simulink model "testHarness"  (R2014b)
settings: Solver=ode15s  StartTime=0.0  StopTime=simTime  RelTol=1e-3
undefined symbols (not defined in the file): amplitude, c1, c11, c12, c13, c14, c15, c16, c17, c18, c19, c2, c20, c21, c22, c23, c24, c25, c3, c4, c5, c6, c7, c8, c9, en_speed
settings Model: Creator=xjin  LastModifiedBy=xjin
settings DataIOCC: LimitDataPoints=off
settings DebuggingCC: UnderspecifiedInitializationDetection=Classic  MergeDetectMultiDrivingBlocksExec=none

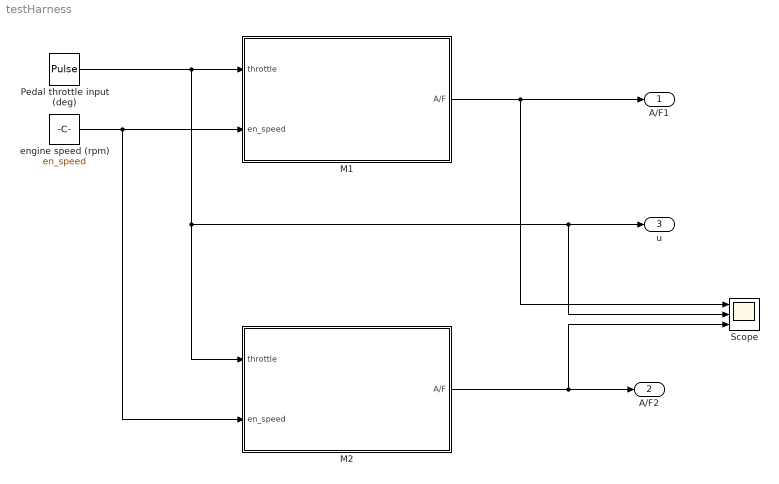
== system testHarness ==
  "M1 " : Subsystem
  M2 : Subsystem
  Pedal throttle input (deg) : DiscretePulseGenerator  PulseType=Time based  Amplitude=amplitude  Period=10  PulseWidth=50  PhaseDelay=3
  Scope : Scope  NumInputPorts=3
      settings: YMin=-5~-5~-5  YMax=5~5~5
  engine speed (rpm) : Constant  Value=en_speed
  A/F1 : Outport
  A/F2 : Outport  Port=2
  u : Outport  Port=3
  wires:
  "M1 "/1(A/F) -> Scope/1, A/F1/1
  engine speed (rpm)/1 -> M2/2(en_speed), "M1 "/2(en_speed)
  Pedal throttle input (deg)/1 -> "M1 "/1(throttle), M2/1(throttle), Scope/2, u/1
  M2/1(A/F) -> Scope/3, A/F2/1

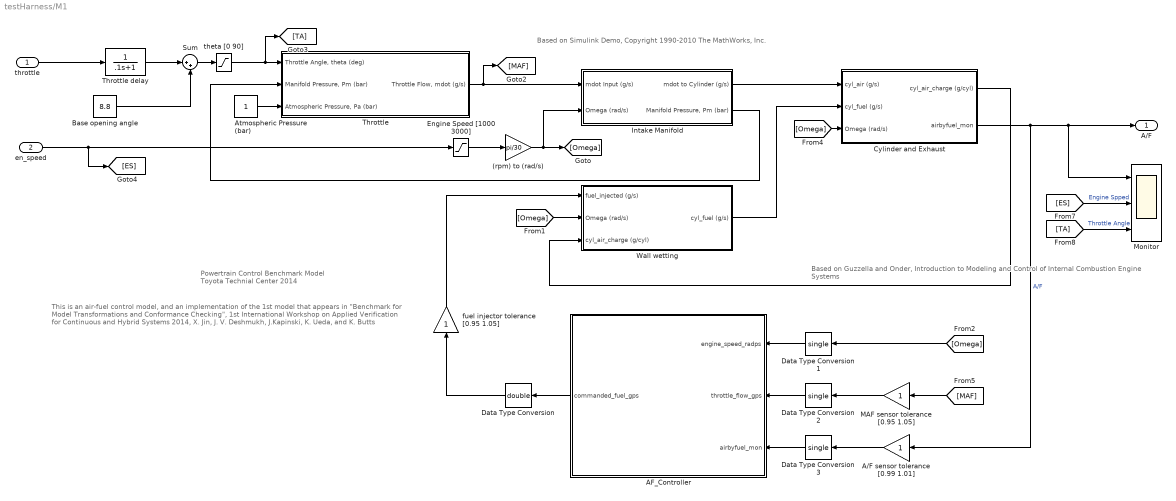
== system testHarness/M1  ==
  note: This is an air-fuel control model, and an implementation of the 1st model that appears in
      | "Benchmark for Model Transformations and Conformance Checking",
      | 1st International Workshop on Applied Verification for Continuous and Hybrid Systems 2014,
      | X. Jin, J. V. Deshmukh, J.Kapinski, K. Ueda, and K. Butts
  note: Powertrain Control Benchmark Model
      | Toyota Technial Center
      | 2014
  note: Based on Simulink Demo, Copyright 1990-2010 The MathWorks, Inc.
  note: Based on Guzzella and Onder, Introduction to Modeling and Control of Internal Combustion Engine Systems
  throttle : Inport
  en_speed : Inport  Port=2
  (rpm) to (rad/s) : Gain  Gain=pi/30
  A/F sensor tolerance [0.99 1.01] : Gain
  AF_Controller : Subsystem  TreatAsAtomicUnit=on
  Atmospheric Pressure (bar) : Constant
  Base opening angle : Constant  Value=8.8
  Cylinder and Exhaust : Subsystem
  Data Type Conversion : DataTypeConversion  OutDataTypeStr=double
  Data Type Conversion1 : DataTypeConversion  OutDataTypeStr=single
  Data Type Conversion2 : DataTypeConversion  OutDataTypeStr=single
  Data Type Conversion3 : DataTypeConversion  OutDataTypeStr=single
  Engine Speed [1000 3000] : Saturate  UpperLimit=3000  LowerLimit=1000
  Intake Manifold : Subsystem
  MAF sensor tolerance [0.95 1.05] : Gain
  Monitor : Scope  NumInputPorts=3
      settings: TimeRange=50  YMin=12.5~2850~5  YMax=20.5~3150~90
  Sum : Sum  Inputs=|++
  Throttle : Subsystem
  Throttle delay : TransferFcn  Denominator=[.1 1]
  Wall wetting : Subsystem
  fuel injector tolerance [0.95 1.05] : Gain
  theta [0 90] : Saturate  UpperLimit=90  LowerLimit=0
  A/F : Outport
  wires:
  (rpm) to (rad/s)/1 -> Intake Manifold/2(Omega (rad/s)), [Omega]
  Data Type Conversion/1 -> fuel injector tolerance [0.95 1.05]/1
  theta [0 90]/1 -> Throttle/1("Throttle Angle, theta (deg)"), [TA]
  Engine Speed [1000 3000]/1 -> (rpm) to (rad/s)/1
  Cylinder and Exhaust/2("airbyfuel_mon ") -> A/F sensor tolerance [0.99 1.01]/1, A/F/1, Monitor/1  "A/F"
  Data Type Conversion2/1 -> AF_Controller/2(throttle_flow_gps)
  Data Type Conversion3/1 -> AF_Controller/3(airbyfuel_mon)
  A/F sensor tolerance [0.99 1.01]/1 -> Data Type Conversion3/1
  [MAF] -> MAF sensor tolerance [0.95 1.05]/1
  Throttle/1("Throttle Flow, mdot (g/s)") -> [MAF], Intake Manifold/1(mdot Input (g/s))
  Intake Manifold/2("Manifold Pressure, Pm (bar)") -> Throttle/2("Manifold Pressure, Pm (bar)")
  Atmospheric Pressure (bar)/1 -> Throttle/3("Atmospheric Pressure, Pa (bar) ")
  Intake Manifold/1(mdot to Cylinder (g/s)) -> Cylinder and Exhaust/1(cyl_air (g/s))
  [Omega] -> Cylinder and Exhaust/3(Omega (rad/s))
  [Omega] -> Wall wetting/2(Omega (rad/s))
  Cylinder and Exhaust/1(cyl_air_charge (g/cyl)) -> Wall wetting/3(cyl_air_charge (g/cyl))
  [Omega] -> Data Type Conversion1/1
  fuel injector tolerance [0.95 1.05]/1 -> Wall wetting/1(fuel_injected (g/s))
  MAF sensor tolerance [0.95 1.05]/1 -> Data Type Conversion2/1
  AF_Controller/1(commanded_fuel_gps) -> Data Type Conversion/1
  Data Type Conversion1/1 -> AF_Controller/1(engine_speed_radps)
  Throttle delay/1 -> Sum/1
  Base opening angle/1 -> Sum/2
  Sum/1 -> theta [0 90]/1
  throttle/1 -> Throttle delay/1
  en_speed/1 -> [ES], Engine Speed [1000 3000]/1
  Wall wetting/1(cyl_fuel (g/s)) -> Cylinder and Exhaust/2(cyl_fuel (g/s))
  [TA] -> Monitor/3  "Throttle Angle"
  [ES] -> Monitor/2  "Engine Spped"

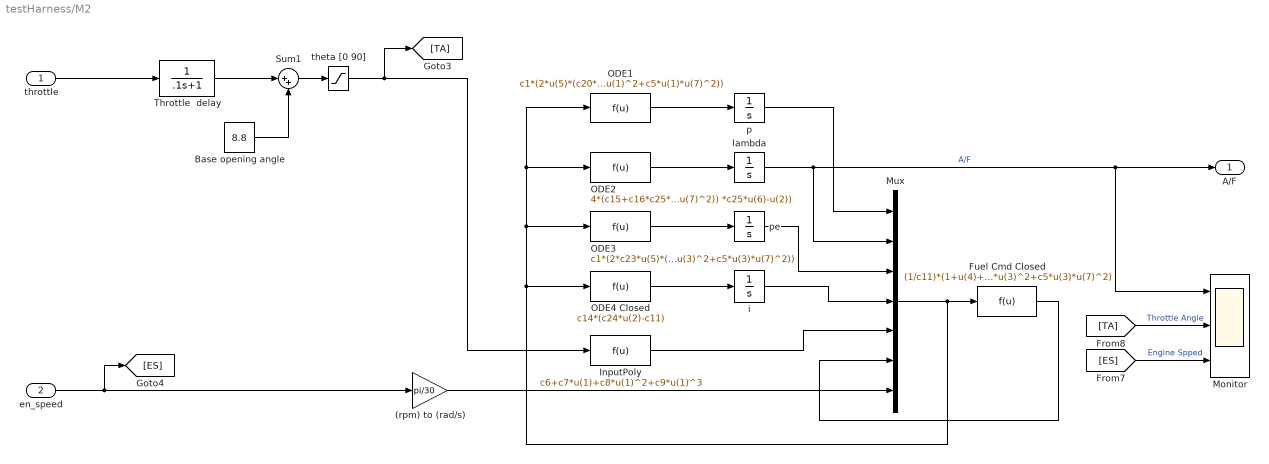
== system testHarness/M2 ==
  throttle : Inport
  en_speed : Inport  Port=2
  (rpm) to (rad/s) : Gain  Gain=pi/30
  Base opening angle : Constant  Value=8.8
  Fuel Cmd Closed : Fcn  Expr=(1/c11)*(1+u(4)+c13*(c24*u(2)-c11))*(c2+c3*u(7)*u(3)+c4*u(7)*u(3)^2+c5*u(3)*u(7)^2)
  InputPoly : Fcn  Expr=c6+c7*u(1)+c8*u(1)^2+c9*u(1)^3
  Monitor : Scope  NumInputPorts=3
      settings: TimeRange=50  YMin=12.5~2850~5  YMax=20.5~3150~90  SaveName=ScopeData2
  Mux : Mux  Inputs=7
  ODE1 : Fcn  Expr=c1*(2*u(5)*(c20*u(1)^2+c21*u(1)+c22) - c12*(c2+c3*u(7)*u(1)+c4*u(7)*u(1)^2+c5*u(1)*u(7)^2))
  ODE2 : Fcn  Expr=4*(c15+c16*c25*u(6)+c17*c25^2*u(6)^2+c18*(c12*(c2+c3*u(7)*u(1)+c4*u(7)*u(1)^2+c5*u(1)*u(7)^2)) +c19*(c12*(c2+c3*u(7)*u(1)+c4*u(7)*u(1)^2+c5*u(1)*u(7)^2)) *c25*u(6)-u(2))
  ODE3 : Fcn  Expr=c1*(2*c23*u(5)*(c20*u(1)^2+c21*u(1)+c22)-(c2+c3*u(7)*u(3)+c4*u(7)*u(3)^2+c5*u(3)*u(7)^2))
  ODE4 Closed : Fcn  Expr=c14*(c24*u(2)-c11)
  Sum1 : Sum  Inputs=|++
  Throttle  delay : TransferFcn  Denominator=[.1 1]
  i : Integrator  InitialCondition=0.017
  lambda : Integrator  InitialCondition=14.7
  p : Integrator  InitialCondition=0.6353
  pe : Integrator  InitialCondition=0.5573
  theta [0 90] : Saturate  UpperLimit=90  LowerLimit=0
  A/F : Outport
  wires:
  ODE1/1 -> p/1
  Mux/1 -> Fuel Cmd Closed/1, ODE1/1, ODE2/1, ODE3/1, ODE4 Closed/1
  InputPoly/1 -> Mux/5
  ODE2/1 -> lambda/1
  p/1 -> Mux/1
  pe/1 -> Mux/3
  i/1 -> Mux/4
  lambda/1 -> Mux/2, Monitor/1, A/F/1  "A/F"
  Fuel Cmd Closed/1 -> Mux/6
  ODE4 Closed/1 -> i/1
  ODE3/1 -> pe/1
  (rpm) to (rad/s)/1 -> Mux/7
  Base opening angle/1 -> Sum1/2
  throttle/1 -> Throttle  delay/1
  Throttle  delay/1 -> Sum1/1
  Sum1/1 -> theta [0 90]/1
  theta [0 90]/1 -> [TA], InputPoly/1
  [TA] -> Monitor/2  "Throttle Angle"
  [ES] -> Monitor/3  "Engine Spped"
  en_speed/1 -> [ES], (rpm) to (rad/s)/1

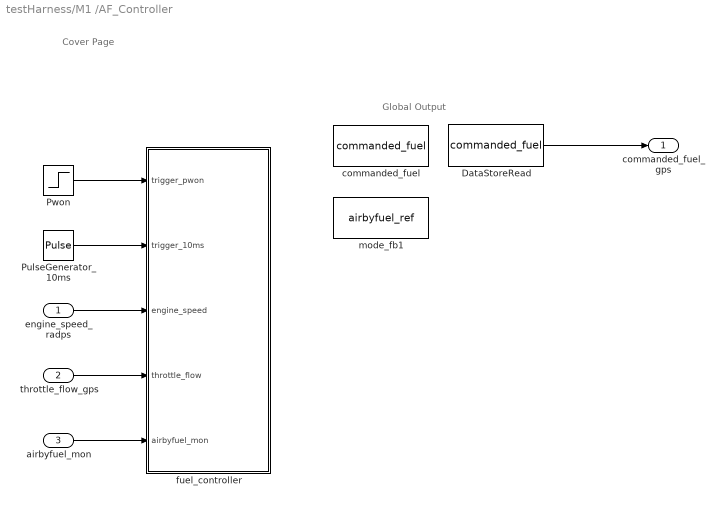
== system testHarness/M1 /AF_Controller ==
  note: Global Output
  note: Cover Page
  engine_speed_radps : Inport
  throttle_flow_gps : Inport  Port=2
  airbyfuel_mon : Inport  Port=3
  DataStoreRead : DataStoreRead  Priority=2  DataStoreName=commanded_fuel
  PulseGenerator_10ms : DiscretePulseGenerator  PulseType=Time based  Period=0.01  PulseWidth=50  PhaseDelay=0.01
  Pwon : Step  Time=0.001  SampleTime=0
  commanded_fuel : DataStoreMemory  DataStoreName=commanded_fuel  InitialValue=0.1726  OutDataTypeStr=single
      settings: AttributesFormatString=commanded_fuel
  fuel_controller : Subsystem  Priority=1  TreatAsAtomicUnit=on
      settings: AttributesFormatString=Priority = %<Priority>
  mode_fb1 : DataStoreMemory  DataStoreName=airbyfuel_ref  InitialValue=14.7  OutDataTypeStr=single
  commanded_fuel_gps : Outport
  wires:
  DataStoreRead/1 -> commanded_fuel_gps/1
  airbyfuel_mon/1 -> fuel_controller/5(airbyfuel_mon)
  throttle_flow_gps/1 -> fuel_controller/4(throttle_flow)
  engine_speed_radps/1 -> fuel_controller/3(engine_speed)
  Pwon/1 -> fuel_controller/1(trigger_pwon)
  PulseGenerator_10ms/1 -> fuel_controller/2(trigger_10ms)

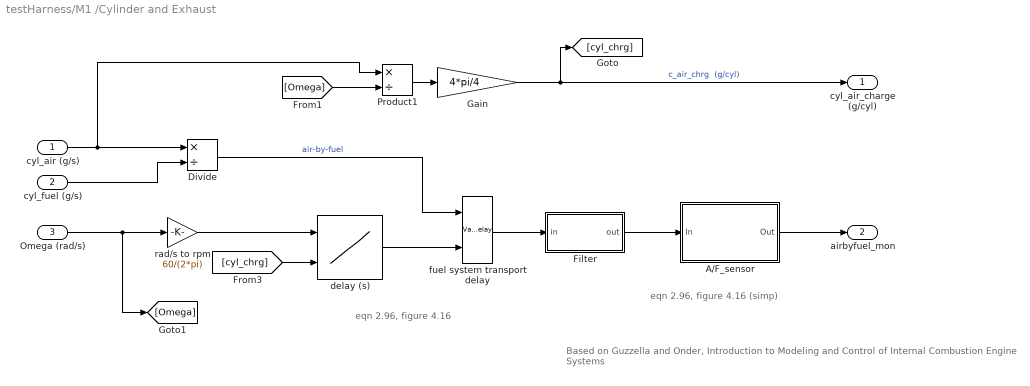
== system testHarness/M1 /Cylinder and Exhaust ==
  note: eqn 2.96, figure 4.16
  note: eqn 2.96, figure 4.16 (simp)
  note: Based on Guzzella and Onder, Introduction to Modeling and Control of Internal Combustion Engine Systems
  cyl_air (g/s) : Inport
  cyl_fuel (g/s) : Inport  Port=2
  Omega (rad/s) : Inport  Port=3
  A/F_sensor : Subsystem
  Divide : Product  Inputs=*/
  Filter : Subsystem
  Gain : Gain  Gain=4*pi/4
  Product1 : Product  Inputs=*/  RndMeth=Zero
  delay (s) : Lookup_n-D  BreakpointsForDimension1=[800,1000,1500,2000,3000]  BreakpointsForDimension2=[0.05,0.15,0.2,0.25]  Table=reshape([0.8,0.6,0.4,0.3,0.2,0.4,0.3,0.2,0.2,0.2,0.3,0.25,0.2,0.2,0.2,0.25,0.2,0.2,0.2,0.2],5,4)  UseLastTableValue=on  RndMeth=Simplest  InputSameDT=on
  fuel system transport delay : VariableTransportDelay  VariableDelayType=Variable transport delay  MaximumDelay=10  InitialOutput=14.7  MaximumPoints=20480
  rad/s to rpm : Gain  Gain=60/(2*pi)
  cyl_air_charge (g/cyl) : Outport
  "airbyfuel_mon " : Outport  Port=2
  wires:
  cyl_air (g/s)/1 -> Divide/1, Product1/1
  [Omega] -> Product1/2
  Product1/1 -> Gain/1
  Gain/1 -> [cyl_chrg], cyl_air_charge (g/cyl)/1  "c_air_chrg  (g/cyl)"
  [cyl_chrg] -> delay (s)/2
  cyl_fuel (g/s)/1 -> Divide/2
  Omega (rad/s)/1 -> [Omega], rad/s to rpm/1
  rad/s to rpm/1 -> delay (s)/1
  delay (s)/1 -> fuel system transport delay/2
  fuel system transport delay/1 -> Filter/1(in)
  Divide/1 -> fuel system transport delay/1  "air-by-fuel"
  Filter/1(out) -> A/F_sensor/1(In)
  A/F_sensor/1(Out) -> "airbyfuel_mon "/1

== system testHarness/M1 /Intake Manifold ==
  note: Intake Manifold Vacuum
  note: Based on Simulink Demo, Copyright 1990-2010 The MathWorks, Inc.
  mdot Input (g/s) : Inport
  Omega (rad/s) : Inport  Port=2
  Gain2 : Gain  Gain=0.9  ParamDataTypeStr=single  OutDataTypeStr=Inherit: Inherit via back propagation  RndMeth=Simplest  SaturateOnIntegerOverflow=on
      settings: AttributesFormatString=pumping tolerance [0.9 1.1]
  Mux : Mux  Inputs=2
  Pumping : Fcn  Expr=-0.366 + 0.08979*u[1]*u[2] - 0.0337*u[2]*u[1]*u[1] + 0.0001*u[1]*u[2]*u[2]
  RT/Vm : Gain  Gain=0.41328  SaturateOnIntegerOverflow=on  OutDataTypeStr=Inherit: Same as input  ParamDataTypeStr=Inherit: Same as input
  Sum : Sum  Inputs=|+-  SaturateOnIntegerOverflow=on  InputSameDT=on  OutDataTypeStr=Inherit: Same as first input
  p0 = 0.543 (bar) : Integrator  InitialCondition=0.7705
  mdot to Cylinder (g/s) : Outport  InitialOutput=0
  "Manifold Pressure, Pm (bar)" : Outport  Port=2  InitialOutput=0
  wires:
  mdot Input (g/s)/1 -> Sum/1
  RT/Vm/1 -> p0 = 0.543 (bar)/1
  Omega (rad/s)/1 -> Mux/2
  Mux/1 -> Pumping/1
  p0 = 0.543 (bar)/1 -> Mux/1, "Manifold Pressure, Pm (bar)"/1
  Sum/1 -> RT/Vm/1
  Pumping/1 -> Gain2/1
  Gain2/1 -> Sum/2, mdot to Cylinder (g/s)/1

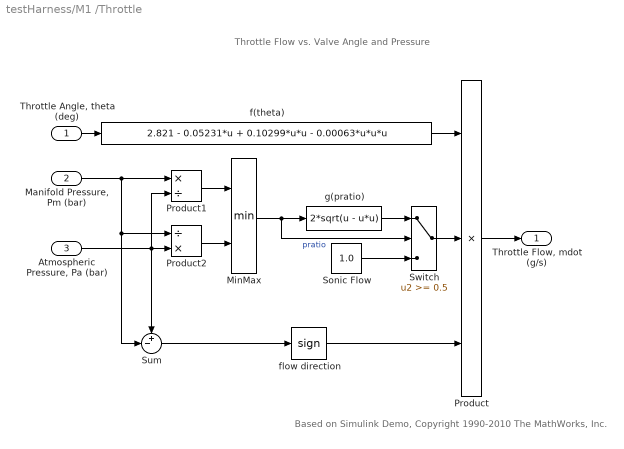
== system testHarness/M1 /Throttle ==
  note: Throttle Flow vs. Valve Angle and Pressure
  note: Based on Simulink Demo, Copyright 1990-2010 The MathWorks, Inc.
  "Throttle Angle, theta (deg)" : Inport
  "Manifold Pressure, Pm (bar)" : Inport  Port=2
  "Atmospheric Pressure, Pa (bar) " : Inport  Port=3
  MinMax : MinMax  Inputs=2  SaturateOnIntegerOverflow=on  InputSameDT=on
  Product : Product  Inputs=3  SaturateOnIntegerOverflow=on  RndMeth=Zero  InputSameDT=on  OutDataTypeStr=Inherit: Same as first input
  Product1 : Product  Inputs=*/  SaturateOnIntegerOverflow=on  RndMeth=Zero  InputSameDT=on  OutDataTypeStr=Inherit: Same as first input
  Product2 : Product  Inputs=/*  SaturateOnIntegerOverflow=on  RndMeth=Zero  InputSameDT=on  OutDataTypeStr=Inherit: Same as first input
  "Sonic Flow " : Constant  Value=1.0
  Sum : Sum  Inputs=+-|  SaturateOnIntegerOverflow=on  InputSameDT=on  OutDataTypeStr=Inherit: Same as first input
  Switch : Switch  Threshold=0.5  SaturateOnIntegerOverflow=on  InputSameDT=on
  f(theta) : Fcn  Expr=2.821 - 0.05231*u + 0.10299*u*u - 0.00063*u*u*u
  flow direction : Signum
  g(pratio) : Fcn  Expr=2*sqrt(u - u*u)
  "Throttle Flow, mdot (g/s)" : Outport  InitialOutput=0
  wires:
  "Manifold Pressure, Pm (bar)"/1 -> Sum/2, Product2/1, Product1/1
  Product2/1 -> MinMax/2
  Product1/1 -> MinMax/1
  "Atmospheric Pressure, Pa (bar) "/1 -> Sum/1, Product2/2, Product1/2
  g(pratio)/1 -> Switch/1
  "Sonic Flow "/1 -> Switch/3
  Switch/1 -> Product/2
  flow direction/1 -> Product/3
  Sum/1 -> flow direction/1
  MinMax/1 -> g(pratio)/1, Switch/2  "pratio"
  "Throttle Angle, theta (deg)"/1 -> f(theta)/1
  Product/1 -> "Throttle Flow, mdot (g/s)"/1
  f(theta)/1 -> Product/1

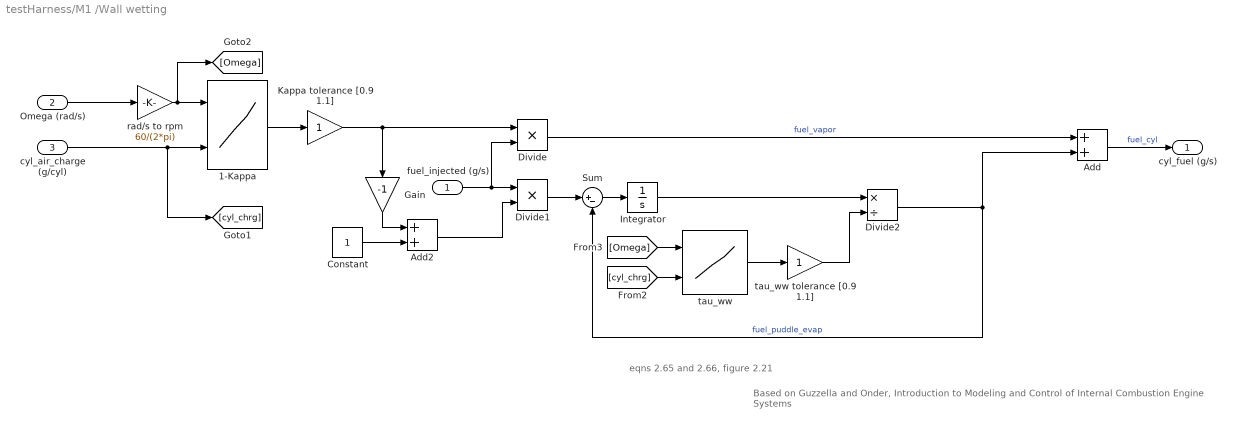
== system testHarness/M1 /Wall wetting ==
  note: eqns 2.65 and 2.66, figure 2.21
  note: Based on Guzzella and Onder, Introduction to Modeling and Control of Internal Combustion Engine Systems
  fuel_injected (g/s) : Inport
  Omega (rad/s) : Inport  Port=2
  cyl_air_charge (g/cyl) : Inport  Port=3
  1-Kappa : Lookup_n-D  BreakpointsForDimension1=[1000,1500,2000,2500,3000]  BreakpointsForDimension2=[.1,.2,.3,.4]  Table=reshape([0.8,.7,.7,.8,.9,.7,.66,.65,.73,.85,.66,.66,.63,.66,.8,.6,.6,.6,.6,.7],5,4)  UseLastTableValue=on  RndMeth=Simplest  InputSameDT=on
  Add : Sum
  Add2 : Sum
  Constant : Constant
  Divide : Product  Inputs=**
  Divide1 : Product  Inputs=**
  Divide2 : Product  Inputs=*/
  Gain : Gain  Gain=-1
  Integrator : Integrator  InitialCondition=.0112
  Kappa tolerance [0.9 1.1] : Gain
  Sum : Sum  Inputs=|+-
  rad/s to rpm : Gain  Gain=60/(2*pi)
  tau_ww : Lookup_n-D  BreakpointsForDimension1=[1000,1500,2000,2500,3000]  BreakpointsForDimension2=[0.1,0.2,0.3,0.4]  Table=reshape([.4,.3,.35,.3,.2,.22,.22,.4,.35,.5,.20,.22,.5,.4,.35,.35,.3,.45,.5,.4],5,4)  UseLastTableValue=on  RndMeth=Simplest  InputSameDT=on
  tau_ww tolerance [0.9 1.1] : Gain
  cyl_fuel (g/s) : Outport
  wires:
  1-Kappa/1 -> Kappa tolerance [0.9 1.1]/1
  fuel_injected (g/s)/1 -> Divide1/1, Divide/2
  Divide/1 -> Add/1  "fuel_vapor"
  Add/1 -> cyl_fuel (g/s)/1  "fuel_cyl"
  Integrator/1 -> Divide2/1
  Divide1/1 -> Sum/1
  Sum/1 -> Integrator/1
  Divide2/1 -> Add/2, Sum/2  "fuel_puddle_evap"
  Add2/1 -> Divide1/2
  [cyl_chrg] -> tau_ww/2
  tau_ww/1 -> tau_ww tolerance [0.9 1.1]/1
  Gain/1 -> Add2/1
  Constant/1 -> Add2/2
  rad/s to rpm/1 -> [Omega], 1-Kappa/1
  Omega (rad/s)/1 -> rad/s to rpm/1
  Kappa tolerance [0.9 1.1]/1 -> Divide/1, Gain/1
  cyl_air_charge (g/cyl)/1 -> 1-Kappa/2, [cyl_chrg]
  [Omega] -> tau_ww/1
  tau_ww tolerance [0.9 1.1]/1 -> Divide2/2

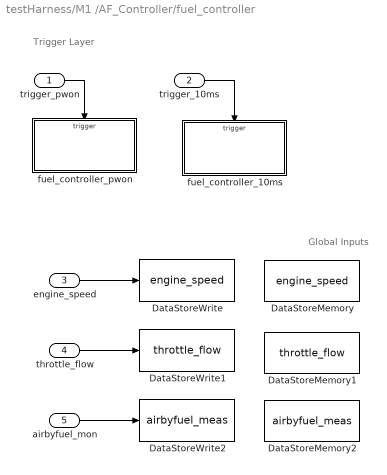
== system testHarness/M1 /AF_Controller/fuel_controller ==
  note: Global Inputs
  note: Trigger Layer
  trigger_pwon : Inport
  trigger_10ms : Inport  Port=2
  engine_speed : Inport  Port=3
  throttle_flow : Inport  Port=4
  airbyfuel_mon : Inport  Port=5
  DataStoreMemory : DataStoreMemory  DataStoreName=engine_speed  OutDataTypeStr=single
      settings: AttributesFormatString=engine speed
  DataStoreMemory1 : DataStoreMemory  DataStoreName=throttle_flow  OutDataTypeStr=single
      settings: AttributesFormatString=throttle flow
  DataStoreMemory2 : DataStoreMemory  DataStoreName=airbyfuel_meas  OutDataTypeStr=single
      settings: AttributesFormatString=lambda_meas
  DataStoreWrite : DataStoreWrite  Priority=1  DataStoreName=engine_speed
  DataStoreWrite1 : DataStoreWrite  Priority=1  DataStoreName=throttle_flow
  DataStoreWrite2 : DataStoreWrite  Priority=1  DataStoreName=airbyfuel_meas
  fuel_controller_10ms : Subsystem  Priority=20  TreatAsAtomicUnit=on
      settings: AttributesFormatString=Priority = %<Priority>
  fuel_controller_pwon : Subsystem  Priority=10  TreatAsAtomicUnit=on
      settings: AttributesFormatString=Priority = %<Priority>
  wires:
  airbyfuel_mon/1 -> DataStoreWrite2/1
  throttle_flow/1 -> DataStoreWrite1/1
  engine_speed/1 -> DataStoreWrite/1
  trigger_10ms/1 -> fuel_controller_10ms/Trigger
  trigger_pwon/1 -> fuel_controller_pwon/Trigger

== system testHarness/M1 /Cylinder and Exhaust/A//F_sensor ==
  In : Inport
  A/F_sensor : Gain  OutDataTypeStr=double
  Filter : Subsystem
  Out : Outport
  wires:
  A/F_sensor/1 -> Out/1
  In/1 -> Filter/1(In)
  Filter/1(Out) -> A/F_sensor/1

== system testHarness/M1 /Cylinder and Exhaust/Filter ==
  in : Inport
  Gain1 : Gain  Gain=10
  Integrator : Integrator  InitialCondition=14.7
  Sum : Sum  Inputs=|+-
  out : Outport
  wires:
  Integrator/1 -> out/1, Sum/2
  in/1 -> Sum/1
  Gain1/1 -> Integrator/1
  Sum/1 -> Gain1/1

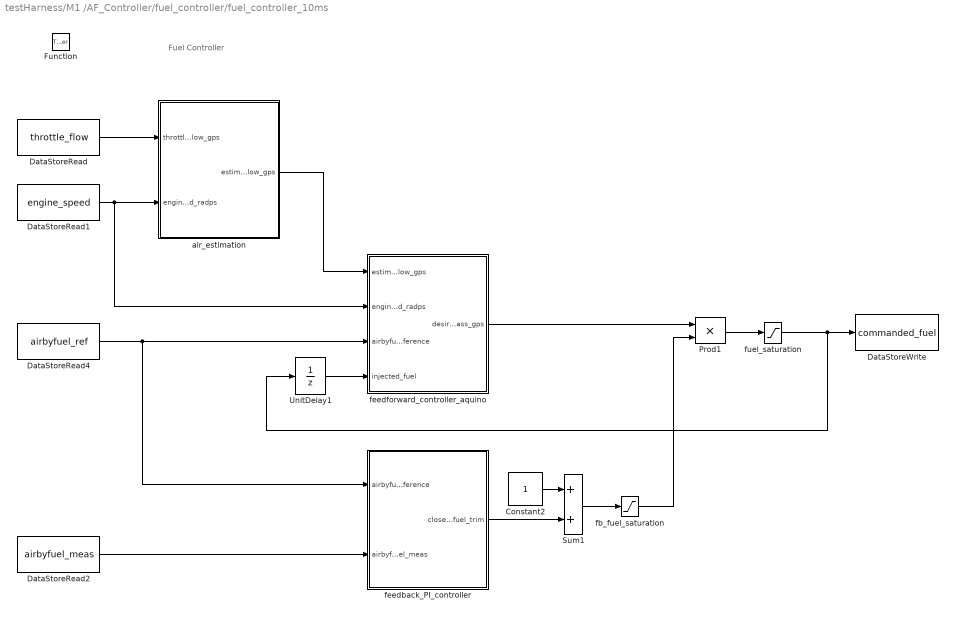
== system testHarness/M1 /AF_Controller/fuel_controller/fuel_controller_10ms ==
  note: Fuel Controller
  Function : TriggerPort
  Constant2 : Constant  OutDataTypeStr=single
  DataStoreRead : DataStoreRead  DataStoreName=throttle_flow
  DataStoreRead1 : DataStoreRead  DataStoreName=engine_speed
  DataStoreRead2 : DataStoreRead  DataStoreName=airbyfuel_meas
  DataStoreRead4 : DataStoreRead  DataStoreName=airbyfuel_ref
  DataStoreWrite : DataStoreWrite  DataStoreName=commanded_fuel
  Prod1 : Product  OutDataTypeStr=Inherit: Inherit via back propagation  RndMeth=Simplest
  Sum1 : Sum  OutDataTypeStr=Inherit: Inherit via back propagation  RndMeth=Simplest  InputSameDT=on
  UnitDelay1 : UnitDelay  SampleTime=-1
      settings: AttributesFormatString=Initial Value = 0
  air_estimation : Subsystem  TreatAsAtomicUnit=on
  fb_fuel_saturation : Saturate  UpperLimit=inf  LowerLimit=0  RndMeth=Round
      settings: AttributesFormatString=y >= 0
  feedback_PI_controller : Subsystem  TreatAsAtomicUnit=on
  feedforward_controller_aquino : Subsystem  TreatAsAtomicUnit=on
  fuel_saturation : Saturate  UpperLimit=5.0  LowerLimit=0.1  RndMeth=Round
      settings: AttributesFormatString=0.1 <=\ncommanded_fuel\n<= 5.0
  wires:
  DataStoreRead4/1 -> feedforward_controller_aquino/3(airbyfuel_reference), feedback_PI_controller/1(airbyfuel_reference)
  Prod1/1 -> fuel_saturation/1
  Constant2/1 -> Sum1/1
  DataStoreRead1/1 -> air_estimation/2(engine_speed_radps), feedforward_controller_aquino/2(engine_speed_radps)
  DataStoreRead/1 -> air_estimation/1(throttle_flow_gps)
  Sum1/1 -> fb_fuel_saturation/1
  fb_fuel_saturation/1 -> Prod1/2
  fuel_saturation/1 -> UnitDelay1/1, DataStoreWrite/1
  DataStoreRead2/1 -> feedback_PI_controller/2(airbyfuel_meas)
  UnitDelay1/1 -> feedforward_controller_aquino/4(injected_fuel)
  feedforward_controller_aquino/1(desired_fuel_mass_gps) -> Prod1/1
  air_estimation/1(estimated_cyl_air_flow_gps) -> feedforward_controller_aquino/1(estimated_cyl_air_flow_gps)
  feedback_PI_controller/1(closed_loop_fuel_trim) -> Sum1/2

== system testHarness/M1 /AF_Controller/fuel_controller/fuel_controller_pwon ==
  Function : TriggerPort
  Constant2 : Constant  Value=0.1726  OutDataTypeStr=single  SampleTime=-1
  Constant3 : Constant  Value=14.7  OutDataTypeStr=single  SampleTime=-1
  DataStoreWrite : DataStoreWrite  DataStoreName=commanded_fuel
  DataStoreWrite2 : DataStoreWrite  DataStoreName=airbyfuel_ref
  wires:
  Constant2/1 -> DataStoreWrite/1
  Constant3/1 -> DataStoreWrite2/1

== system testHarness/M1 /Cylinder and Exhaust/A//F_sensor/Filter ==
  In : Inport
  Gain : Gain  Gain=50
  Integrator : Integrator  InitialCondition=14.7
  Sum : Sum  Inputs=|+-
  Out : Outport
  wires:
  Integrator/1 -> Out/1, Sum/2
  In/1 -> Sum/1
  Gain/1 -> Integrator/1
  Sum/1 -> Gain/1

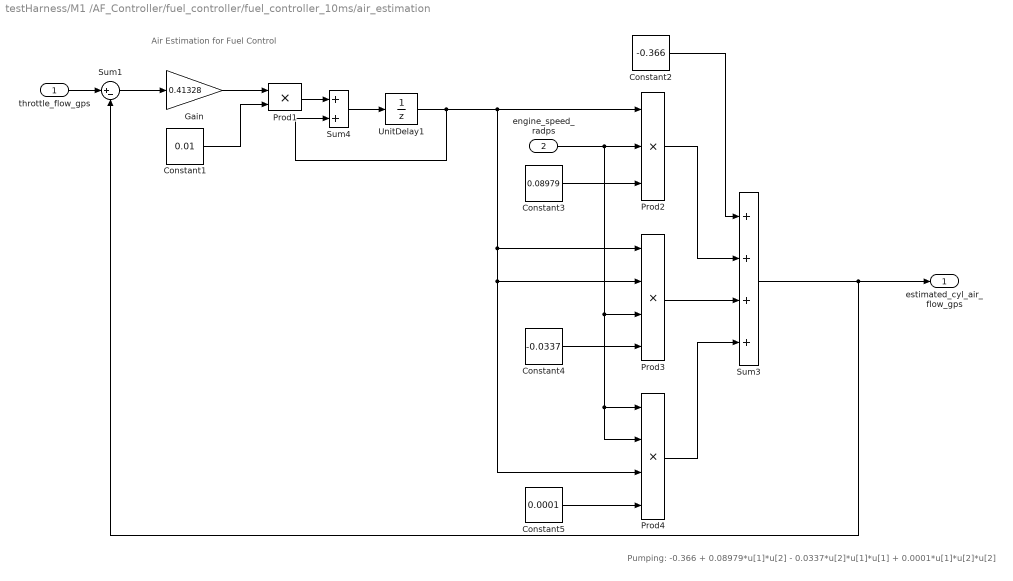
== system testHarness/M1 /AF_Controller/fuel_controller/fuel_controller_10ms/air_estimation ==
  note: Air Estimation for Fuel Control
  note: Pumping: -0.366 + 0.08979*u[1]*u[2] - 0.0337*u[2]*u[1]*u[1] + 0.0001*u[1]*u[2]*u[2]
  throttle_flow_gps : Inport
  engine_speed_radps : Inport  Port=2
  Constant1 : Constant  Value=0.01  OutDataTypeStr=single  SampleTime=-1
      settings: AttributesFormatString=Sample Time (s)
  Constant2 : Constant  Value=-0.366  OutDataTypeStr=single  SampleTime=-1
  Constant3 : Constant  Value=0.08979  OutDataTypeStr=single  SampleTime=-1
  Constant4 : Constant  Value=-0.0337  OutDataTypeStr=single  SampleTime=-1
  Constant5 : Constant  Value=0.0001  OutDataTypeStr=single  SampleTime=-1
  Gain : Gain  Gain=0.41328  ParamDataTypeStr=single  OutDataTypeStr=Inherit: Inherit via back propagation  RndMeth=Simplest  SaturateOnIntegerOverflow=on
      settings: AttributesFormatString=RT/Vm
  Prod1 : Product  OutDataTypeStr=Inherit: Inherit via back propagation  RndMeth=Simplest
  Prod2 : Product  Inputs=3  OutDataTypeStr=Inherit: Inherit via back propagation  RndMeth=Simplest
  Prod3 : Product  Inputs=4  OutDataTypeStr=Inherit: Inherit via back propagation  RndMeth=Simplest
  Prod4 : Product  Inputs=4  OutDataTypeStr=Inherit: Inherit via back propagation  RndMeth=Simplest
  Sum1 : Sum  Inputs=|+-  OutDataTypeStr=Inherit: Inherit via back propagation  RndMeth=Simplest  InputSameDT=on
  Sum3 : Sum  Inputs=++++  OutDataTypeStr=Inherit: Inherit via back propagation  RndMeth=Simplest  InputSameDT=on
  Sum4 : Sum  OutDataTypeStr=Inherit: Inherit via back propagation  RndMeth=Simplest  InputSameDT=on
  UnitDelay1 : UnitDelay  InitialCondition=0.825  SampleTime=-1
      settings: AttributesFormatString=p0 = %<InitialCondition> (bar)
  estimated_cyl_air_flow_gps : Outport
  wires:
  Sum3/1 -> Sum1/2, estimated_cyl_air_flow_gps/1
  Constant5/1 -> Prod4/4
  Constant4/1 -> Prod3/4
  Constant3/1 -> Prod2/3
  engine_speed_radps/1 -> Prod4/2, Prod4/1, Prod3/3, Prod2/2
  Prod4/1 -> Sum3/4
  Prod3/1 -> Sum3/3
  Prod2/1 -> Sum3/2
  Constant2/1 -> Sum3/1
  throttle_flow_gps/1 -> Sum1/1
  Sum1/1 -> Gain/1
  Gain/1 -> Prod1/1
  UnitDelay1/1 -> Sum4/2, Prod4/3, Prod3/2, Prod3/1, Prod2/1
  Prod1/1 -> Sum4/1
  Constant1/1 -> Prod1/2
  Sum4/1 -> UnitDelay1/1

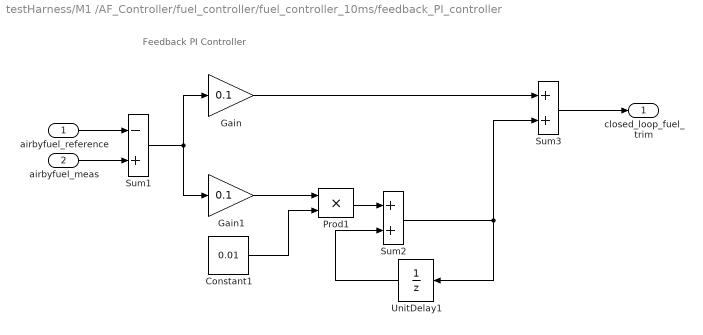
== system testHarness/M1 /AF_Controller/fuel_controller/fuel_controller_10ms/feedback_PI_controller ==
  note: Feedback PI Controller
  airbyfuel_reference : Inport
  airbyfuel_meas : Inport  Port=2
  Constant1 : Constant  Value=0.01  OutDataTypeStr=single  SampleTime=-1
      settings: AttributesFormatString=Sample Time [s]
  Gain : Gain  Gain=0.1  ParamDataTypeStr=single  OutDataTypeStr=Inherit: Inherit via back propagation  RndMeth=Simplest  SaturateOnIntegerOverflow=on
      settings: AttributesFormatString=Proportional Gain
  Gain1 : Gain  Gain=0.1  ParamDataTypeStr=single  OutDataTypeStr=Inherit: Inherit via back propagation  RndMeth=Simplest  SaturateOnIntegerOverflow=on
      settings: AttributesFormatString=Integral Gain
  Prod1 : Product  OutDataTypeStr=Inherit: Inherit via back propagation  RndMeth=Simplest
  Sum1 : Sum  Inputs=-+  OutDataTypeStr=Inherit: Inherit via back propagation  RndMeth=Simplest  InputSameDT=on
  Sum2 : Sum  OutDataTypeStr=Inherit: Inherit via back propagation  RndMeth=Simplest  InputSameDT=on
  Sum3 : Sum  OutDataTypeStr=Inherit: Inherit via back propagation  RndMeth=Simplest  InputSameDT=on
  UnitDelay1 : UnitDelay  SampleTime=-1
      settings: AttributesFormatString=Initial Value = 0
  closed_loop_fuel_trim : Outport
  wires:
  Sum3/1 -> closed_loop_fuel_trim/1
  airbyfuel_reference/1 -> Sum1/1
  airbyfuel_meas/1 -> Sum1/2
  Gain/1 -> Sum3/1
  Sum1/1 -> Gain1/1, Gain/1
  Gain1/1 -> Prod1/1
  Sum2/1 -> UnitDelay1/1, Sum3/2
  Constant1/1 -> Prod1/2
  Prod1/1 -> Sum2/1
  UnitDelay1/1 -> Sum2/2

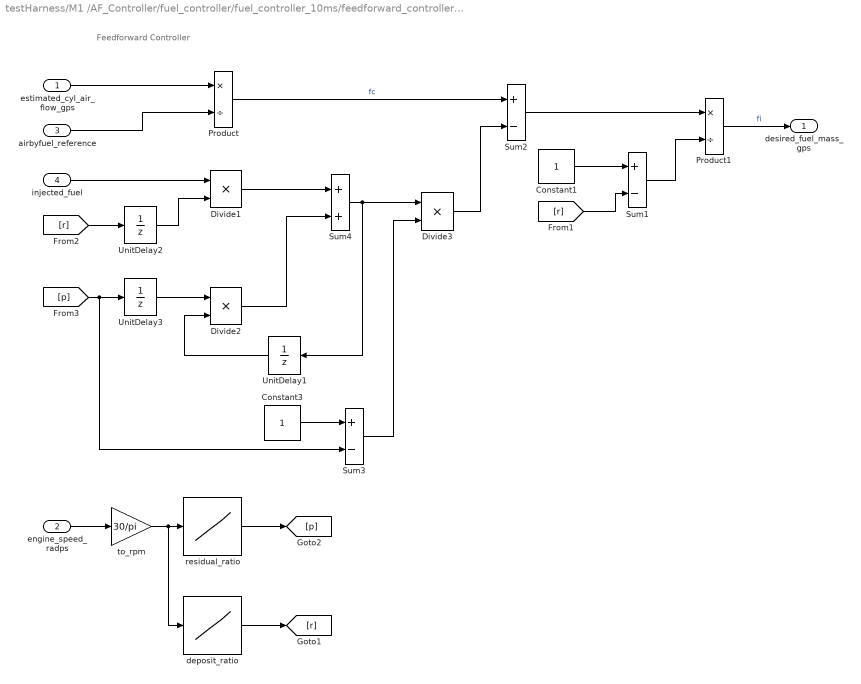
== system testHarness/M1 /AF_Controller/fuel_controller/fuel_controller_10ms/feedforward_controller_aquino ==
  note: Feedforward Controller
  estimated_cyl_air_flow_gps : Inport
  engine_speed_radps : Inport  Port=2
  airbyfuel_reference : Inport  Port=3
  injected_fuel : Inport  Port=4
  Constant1 : Constant  OutDataTypeStr=single  SampleTime=-1
  Constant3 : Constant  OutDataTypeStr=single  SampleTime=-1
  Divide1 : Product  Inputs=**
  Divide2 : Product  Inputs=**
  Divide3 : Product  Inputs=**
  Product : Product  Inputs=*/  RndMeth=Simplest  SaturateOnIntegerOverflow=on  OutDataTypeStr=Inherit: Same as first input
  Product1 : Product  Inputs=*/  RndMeth=Simplest  SaturateOnIntegerOverflow=on  OutDataTypeStr=Inherit: Same as first input
  Sum1 : Sum  Inputs=+-  OutDataTypeStr=Inherit: Inherit via back propagation  RndMeth=Simplest  InputSameDT=on
  Sum2 : Sum  Inputs=+-  OutDataTypeStr=Inherit: Inherit via back propagation  RndMeth=Simplest  InputSameDT=on
  Sum3 : Sum  Inputs=+-  OutDataTypeStr=Inherit: Inherit via back propagation  RndMeth=Simplest  InputSameDT=on
  Sum4 : Sum  OutDataTypeStr=Inherit: Inherit via back propagation  RndMeth=Simplest  InputSameDT=on
  UnitDelay1 : UnitDelay  SampleTime=-1
      settings: AttributesFormatString=Initial Value = 0
  UnitDelay2 : UnitDelay  SampleTime=-1
      settings: AttributesFormatString=Initial Value = 0
  UnitDelay3 : UnitDelay  SampleTime=-1
      settings: AttributesFormatString=Initial Value = 0
  deposit_ratio : Lookup_n-D  NumberOfTableDimensions=1  BreakpointsForDimension1=[1000, 2000, 3000]  Table=[0.4, 0.65, 0.5]  ExtrapMethod=Clip  InternalRulePriority=Speed  RndMeth=Simplest  InputSameDT=on
  residual_ratio : Lookup_n-D  NumberOfTableDimensions=1  BreakpointsForDimension1=[1000, 2000, 3000]  Table=[0.5, 0.95, 0.9]  ExtrapMethod=Clip  InternalRulePriority=Speed  RndMeth=Simplest  InputSameDT=on
  to_rpm : Gain  Gain=30/pi
  desired_fuel_mass_gps : Outport
  wires:
  estimated_cyl_air_flow_gps/1 -> Product/1
  airbyfuel_reference/1 -> Product/2
  Constant3/1 -> Sum3/1
  [p] -> Sum3/2, UnitDelay3/1
  Constant1/1 -> Sum1/1
  [r] -> Sum1/2
  Sum1/1 -> Product1/2
  Product1/1 -> desired_fuel_mass_gps/1  "fi"
  Product/1 -> Sum2/1  "fc"
  injected_fuel/1 -> Divide1/1
  [r] -> UnitDelay2/1
  Divide1/1 -> Sum4/1
  Divide2/1 -> Sum4/2
  Sum4/1 -> Divide3/1, UnitDelay1/1
  UnitDelay1/1 -> Divide2/2
  Sum3/1 -> Divide3/2
  Divide3/1 -> Sum2/2
  Sum2/1 -> Product1/1
  UnitDelay2/1 -> Divide1/2
  UnitDelay3/1 -> Divide2/1
  engine_speed_radps/1 -> to_rpm/1
  to_rpm/1 -> residual_ratio/1, deposit_ratio/1
  deposit_ratio/1 -> [r]
  residual_ratio/1 -> [p]
